simulink model "LAB1"  (R2020b)
settings: Solver=VariableStepAuto  StartTime=0.0  StopTime=10.0  RelTol=1e-3
undefined symbols (not defined in the file): magnitude
settings Model: Creator=dssan  LastModifiedBy=dssan

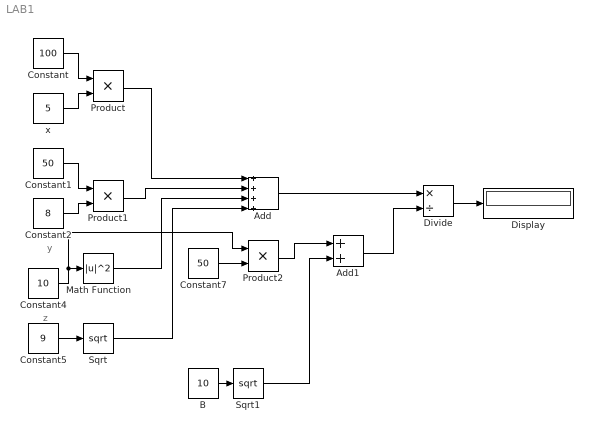
== system LAB1 ==
  note: z
  note: y
  Add : Sum  Inputs=++++
  Add1 : Sum
  B : Constant  Value=10
  Constant : Constant  Value=100
  Constant1 : Constant  Value=50
  Constant2 : Constant  Value=8
  Constant4 : Constant  Value=10
  Constant5 : Constant  Value=9
  Constant7 : Constant  Value=50
  Display : Display
  Divide : Product  Inputs=*/
  Math Function : Math  Operator=magnitude^2  SaturateOnIntegerOverflow=on
  Product : Product
  Product1 : Product
  Product2 : Product
  Sqrt : Sqrt  SaturateOnIntegerOverflow=on
  Sqrt1 : Sqrt  SaturateOnIntegerOverflow=on
  x : Constant  Value=5
  wires:
  Constant/1 -> Product/1
  x/1 -> Product/2
  Constant1/1 -> Product1/1
  Constant2/1 -> Product1/2
  Constant4/1 -> Product2/1, Math Function/1
  Product/1 -> Add/1
  Product1/1 -> Add/2
  Math Function/1 -> Add/3
  Sqrt/1 -> Add/4
  Constant5/1 -> Sqrt/1
  Add/1 -> Divide/1
  B/1 -> Sqrt1/1
  Sqrt1/1 -> Add1/2
  Constant7/1 -> Product2/2
  Product2/1 -> Add1/1
  Add1/1 -> Divide/2
  Divide/1 -> Display/1
